simulink library "myLib_CustomBoolean"  (R2021b)
settings: Solver=VariableStepAuto  StartTime=0.0  StopTime=10.0  RelTol=1e-3
undefined symbols (not defined in the file or in its folder): get, gray, res
libraries: dspobslib x1
settings Model: Creator=abayles  LastModifiedBy=matt
settings SolverCC: AlgebraicLoopSolver=TrustRegion
settings DebuggingCC: SFMachineParentedDataDiag=warning

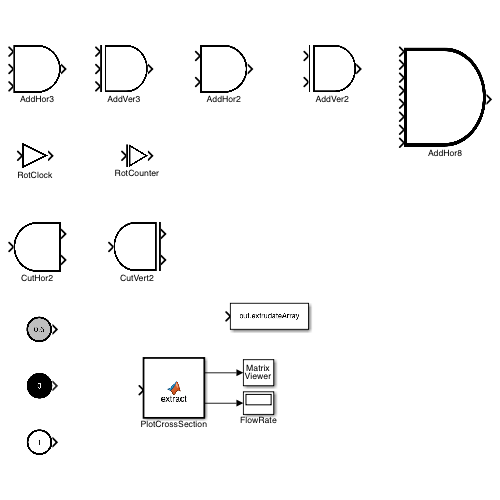
[thumbnail: Simulink's stored preview of the top-level diagram]
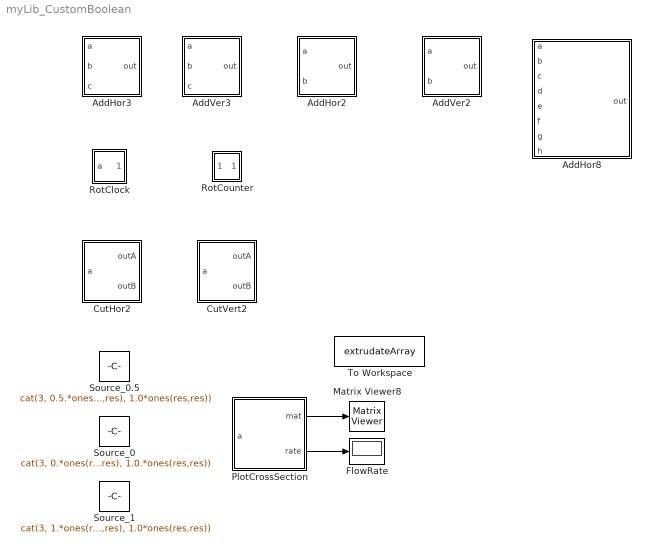
== system myLib_CustomBoolean ==
  AddHor2 : MATLAB Function  TreatAsAtomicUnit=on
  AddHor3 : MATLAB Function  TreatAsAtomicUnit=on
  AddHor8 : MATLAB Function  TreatAsAtomicUnit=on
  AddVer2 : MATLAB Function  TreatAsAtomicUnit=on
  AddVer3 : MATLAB Function  TreatAsAtomicUnit=on
  CutHor2 : MATLAB Function  TreatAsAtomicUnit=on
  CutVert2 : MATLAB Function  TreatAsAtomicUnit=on
  FlowRate : Display
  Matrix Viewer8 : dspobslib/Matrix Viewer  ImageParams=off  CMapStr=gray(3)  AxisColorbar=on  AxisParams=off  AxisOrigin=Upper left corner  AxisTickMode=User-defined  XTickRange=[0 1]  YTickRange=[0 1]  XLabel=X-axis  YLabel=Y-axis  ZLabel=Z-axis  FigPos=get(0,'defaultfigureposition')  AxisZoom=off
      settings: SourceProductBaseCode=DS  YMin=0  YMax=1
  PlotCrossSection : MATLAB Function  TreatAsAtomicUnit=on
  RotClock : MATLAB Function  TreatAsAtomicUnit=on
  RotCounter : MATLAB Function  TreatAsAtomicUnit=on
  Source_0 : Constant  Value=cat(3, 0.*ones(res,res), 1.0.*ones(res,res))  VectorParams1D=off
      mask Display:
      | % Use "Edit Image" on toolstrip to change.
      | % Insert file path below.
      | image('/Users/matt/Documents/MATLAB/UD/AdvectiveAssembly_BooleanSimulink/AdvectiveAssembly_BooleanSimulink/Examples_202112/Manuscripts/Matt-Code_v20220330/PicturesForMasks/source0.png');
  Source_0.5 : Constant  Value=cat(3, 0.5.*ones(res,res), 1.0*ones(res,res))  VectorParams1D=off
      mask Display:
      | % Use "Edit Image" on toolstrip to change.
      | % Insert file path below.
      | image('/Users/matt/Documents/MATLAB/UD/AdvectiveAssembly_BooleanSimulink/AdvectiveAssembly_BooleanSimulink/Examples_202112/Manuscripts/Matt-Code_v20220330/PicturesForMasks/source0_5.png');
  Source_1 : Constant  Value=cat(3, 1.*ones(res,res), 1.0*ones(res,res))  VectorParams1D=off
      mask Display:
      | % Use "Edit Image" on toolstrip to change.
      | % Insert file path below.
      | image('/Users/matt/Documents/MATLAB/UD/AdvectiveAssembly_BooleanSimulink/AdvectiveAssembly_BooleanSimulink/Examples_202112/Manuscripts/Matt-Code_v20220330/PicturesForMasks/source1.png');
  To Workspace : ToWorkspace  VariableName=extrudateArray  SampleTime=51
  wires:
  PlotCrossSection/1(mat) -> Matrix Viewer8/1
  PlotCrossSection/2(rate) -> FlowRate/1

== matlab function myLib_CustomBoolean/AddHor2 ==
  data: a input; out output; b input
function out = add2Hor(a, b)

== matlab function myLib_CustomBoolean/AddVer2 ==
  data: a input; out output; b input
function out = add2Ver(a,b)
%% Version and general code information
%Add Vertical V 1.0 Updated 2022-04-07
% Inputs 
    % Two 3D arrays
% Outputs
    %One 3D array
    %First 2D array (out(:,:,1)) contains the pattern.
    %last element contains the flow rate (out(:,:,2)), should be a
    %constant.

%% Determining preliminary variables
resolution = size(a,1); %Calculates resolution based off of the first dimension (# of rows) of a.
numMatrices = nargin; %Determines the number of matrices based off of the number of input arguments, two.
allMat = nan(resolution,resolution, 2*numMatrices); % Determines the total 3D array size based off the provided resolution and number of matrices. For this case the dimensions are (resolution, resolution, 4).
allMat(:,:, 1:2) = a; %Assigns all the rows and columns of the 1st and 2nd third dimension of the supplied a array to allMat. The 1st and 2nd will contain the pattern and flow rate arrays respectively.
allMat(:,:, 3:4) = b; %Assigns all the rows and columns of the 1st and 2nd third dimension of the supplied b array to allMat. The 3rd and 4th will contain the pattern and flow rate arrays of b respectively.

%% Flow rate calculation
flowRate = nan(numMatrices,1); %Create an empty vector that has numMatrices in rows (2) and 1 column.

for i = 1:numMatrices % Loop from 1 to the final number of matrices two.
    flowRate(i) = allMat(1,1,2*i); % Obtains the flow rate of each entering stream. Upon each loop iteration "grab" the 1st row, 1st column, and 2*i position in the array and assign it to the i'th spot in the flow rate vector. 
end

totalFlowRate = sum(flowRate); % Calculates the total flowrate by adding all entries in the flow rate vector.

%% Constructing the pattern matrix
reduceA = imresize(a(:,:,1),[resolution*flowRate(1)/totalFlowRate, resolution],'nearest'); % Take the pattern a(:,:,1) and resize into the specified dimensions based of the fraction of total flow rate (rows) and resolution (columns). Weights each of the matrices based on their respective flow rates (flowrate(1)).  
reduceB = imresize(b(:,:,1),[resolution*flowRate(2)/totalFlowRate, resolution],'nearest'); % Take the pattern b(:,:,1) and resize into the specified dimensions based of the fraction of total flow rate (rows) and resolution (columns). Weights each of the matrices based on their respective flow rates (flowrate(2)).  
addMatrix = [reduceA; reduceB]; % Vertically concatenates the matrices together.
addMatrix = imresize(addMatrix,[resolution, resolution],'nearest'); %Resize the image to the desired resolution dimensions. 
%% Predefining output variables
out = a; %Assigns the correct dimensions for the output variable.
out(:,:,1) = addMatrix; %Assigns the added pattern array to the output variable.
out(:,:,2) = totalFlowRate.*ones(resolution,resolution); %Defines the flow rate 2D array out(:,:,2). Calculates the new flow rate array using the total flow rate multiplied by a ones matrix of size based on the supplied resolution.

== matlab function myLib_CustomBoolean/AddHor8 ==
  data: a input; out output; b input; c input; d input; e input; f input; g input; h input
function out = add8Hor(a,b,c,d,e,f,g,h)
%% Version and general code information
%Horizontal Addition V 1.0 Updated 2022-04-07
% Inputs
    %Eight 3D arrays
% Outputs
    %3D array 
    % First 2D array (out(:,:,1)) contains the pattern
    %Last element (out(:,:,2)) contains the flow rates, should be a
    %constant

%% Determine preliminary variabes
resolution = size(a,1); %Calculates resolution based off of the first dimension (# of rows) of a
numMatrices = nargin; %Determines the number of matrices based off of the number of input arguments, eight.
allMat = nan(resolution,resolution, 2*numMatrices); % Determines the total 3D array size based off the provided resolution and number of matrices. For this case the dimensions are (resolution, resolution, 16).
allMat(:,:, 1:2) = a; %Assigns all the rows and columns of the 1st and 2nd third dimension of the supplied a array to allMat. The 1st and 2nd will contain the pattern and flow rate arrays of a respectively.
allMat(:,:, 3:4) = b; %Assigns all the rows and columns of the 1st and 2nd third dimension of the supplied b array to allMat. The 3rd and 4th will contain the pattern and flow rate arrays of b respectively.
allMat(:,:, 5:6) = c; %Assigns all the rows and columns of the 1st and 2nd third dimension of the supplied c array to allMat. The 5th and 6th will contain the pattern and flow rate arrays of c respectively.
allMat(:,:, 7:8) = d; %Assigns all the rows and columns of the 1st and 2nd third dimension of the supplied d array to allMat. The 7th and 8th will contain the pattern and flow rate arrays of d respectively.
allMat(:,:, 9:10) = e; %Assigns all the rows and columns of the 1st and 2nd third dimension of the supplied e array to allMat. The 9th and 10th will contain the pattern and flow rate arrays of e respectively.
allMat(:,:, 11:12) = f; %Assigns all the rows and columns of the 1st and 2nd third dimension of the supplied f array to allMat. The 11th and 12th will contain the pattern and flow rate arrays of f respectively.
allMat(:,:, 13:14) = g; %Assigns all the rows and columns of the 1st and 2nd third dimension of the supplied g array to allMat. The 11th and 12th will contain the pattern and flow rate arrays of g respectively.
allMat(:,:, 15:16) = h; %Assigns all the rows and columns of the 1st and 2nd third dimension of the supplied a array to allMat. The 15th and 16th will contain the pattern and flow rate arrays of h respectively.

%% Flow rate calculation
flowRate = nan(numMatrices,1); %Create an empty vector that has numMatrices in rows (8) and 1 column.
for i = 1:numMatrices % Loop from 1 to the final number of matrices 8.
    flowRate(i) = allMat(1,1,2*i); % Obtains the flow rate of each entering stream. Upon each loop iteration "grab" the 1st row, 1st column, and 2*i position in the array and assign it to the i'th spot in the flow rate vector. 
end
totalFlowRate = sum(flowRate); % Calculates the total flowrate by adding all entries in the flow rate vector.
%% Constructing the combined pattern matrix
reduceA = imresize(a(:,:,1),[resolution,resolution*flowRate(1)/totalFlowRate],'nearest'); % Take the pattern a(:,:,1) and resize into the specified dimensions based of the fraction of total flow rate (rows) and resolution (columns). Weights each of the matrices based on their respective flow rates (flowrate(1)).  
reduceB = imresize(b(:,:,1),[resolution,resolution*flowRate(2)/totalFlowRate],'nearest'); % Take the pattern b(:,:,1) and resize into the specified dimensions based of the fraction of total flow rate (rows) and resolution (columns). Weights each of the matrices based on their respective flow rates (flowrate(2)).  
reduceC = imresize(c(:,:,1),[resolution,resolution*flowRate(3)/totalFlowRate],'nearest'); % Take the pattern c(:,:,1) and resize into the specified dimensions based of the fraction of total flow rate (rows) and resolution (columns). Weights each of the matrices based on their respective flow rates (flowrate(3)).  
reduceD = imresize(d(:,:,1),[resolution,resolution*flowRate(4)/totalFlowRate],'nearest'); % Take the pattern d(:,:,1) and resize into the specified dimensions based of the fraction of total flow rate (rows) and resolution (columns). Weights each of the matrices based on their respective flow rates (flowrate(4)).  
reduceE = imresize(e(:,:,1),[resolution,resolution*flowRate(5)/totalFlowRate],'nearest'); % Take the pattern e(:,:,1) and resize into the specified dimensions based of the fraction of total flow rate (rows) and resolution (columns). Weights each of the matrices based on their respective flow rates (flowrate(5)).  
reduceF = imresize(f(:,:,1),[resolution,resolution*flowRate(6)/totalFlowRate],'nearest'); % Take the pattern f(:,:,1) and resize into the specified dimensions based of the fraction of total flow rate (rows) and resolution (columns).  Weights each of the matrices based on their respective flow rates (flowrate(6)).  
reduceG = imresize(g(:,:,1),[resolution,resolution*flowRate(7)/totalFlowRate],'nearest'); % Take the pattern g(:,:,1) and resize into the specified dimensions based of the fraction of total flow rate (rows) and resolution (columns). Weights each of the matrices based on their respective flow rates (flowrate(7)).  
reduceH = imresize(h(:,:,1),[resolution,resolution*flowRate(8)/totalFlowRate],'nearest'); % Take the pattern h(:,:,1) and resize into the specified dimensions based of the fraction of total flow rate (rows) and resolution (columns). Weights each of the matrices based on their respective flow rates (flowrate(8)).  


addMatrix = [reduceH,reduceG,reduceF,reduceE, reduceD,reduceC, reduceB, reduceA]; % Horizontally concatenates the matrices together. The point of view is from the perspective of the extrudate.
addMatrix = imresize(addMatrix,[resolution, 2.*resolution],'nearest'); %Resize the image to the desired resolution dimensions. 


%% Predefining output variables

out = [a,a]; %Assigns the correct dimensions for the output variable.
 
out(:,:,1) = addMatrix; %Assigns the added pattern array to the output variable.
out(:,:,2) = totalFlowRate.*ones(resolution,2.*resolution); %Defines the flow rate 2D array out(:,:,2). Calculates the new flow rate array using the total flow rate multiplied by a ones matrix of size based on the supplied resolution.

== matlab function myLib_CustomBoolean/RotClock ==
  data: a input; out output
function out = rotClock(a)
%% Version and general code information. 
%Rotating Clockwise Block V 1.0 Updated 2022-04-07
% Inputs:
    %3D array with pattern a(:,:,1) and flow rate a(:,:2)
%Outputs:
    %3D array
            %First 2D array (i.e., out(:,:,1)) contains the pattern
            %Last element contains the flow rate (i.e. out(:,:,2)), should be a
            %constant value.
%% Determine preliminary variables
resolution = size(a,1); %Calculates resolution based off of the first dimension (# of rows) of a.

%% Predefining output variables
out = a; %Assigns the correct dimensions for the output variable
out(:,:,1) = rot90(rot90(rot90(a(:,:,1)))); %Rotates the pattern array (a(:,:,1)) 270 degrees counterclockwise ---> 90 degrees clockwise
out(:,:,2) = a(1,1,2).*ones(resolution,resolution); % Defines the flow rate 2D array a(:,:,2)

== matlab function myLib_CustomBoolean/RotCounter ==
  data: a input; out output
function out = rotCounter(a)
%% Version and general code information
%Rotating Counter Clockwise V 1.0 Updated 2022-31-3
% Inputs:
    %3D array with pattern a(:,:,1) and flow rate a(:,:2)
%Outputs:
    %3D array
        %First 2D array (i.e., out(:,:,1)) contains the pattern
        %Last element contains the flow rate (i.e. out(:,:,2)), should be a
        %constant value.
%% Determining prelminary variables
resolution = size(a,1); %Calculates resolution based off of the first dimension (# of rows) of a.

%% Predefining output variables
out = a; %Assigns the correct dimensions for the output variable
out(:,:,1) = rot90(a(:,:,1)); % Rotates the pattern array a(:,:,1)90 degrees counterclockwise
out(:,:,2) = a(1,1,2).*ones(resolution,resolution); % Defines the flow rate 2D array a(:,:,2)

== matlab function myLib_CustomBoolean/AddHor3 ==
  data: a input; out output; b input; c input
function out = add3Hor(a, b, c)

== matlab function myLib_CustomBoolean/CutHor2 ==
  data: a input; outA output; outB output
function [outA, outB] = cutHor(a)
%% Version and general code information
%Cut Horizontal V 1.0 Updated 2022-04-07
% Inputs 
    % One 3D array
% Outputs
    %Two 3D arrays
    %First 2D array (out(:,:,1)) contains the pattern.
    %last element contains the flow rate (out(:,:,2)), should be a
    %constant.

%% Determining preliminary variables
resolution = size(a,1); %Calculates resolution based off of the first dimension (# of rows) of a.
numMatrices = nargin; %Calculates the number of matrices based off  the supplied input arguments, one. 
numOutMatrices = nargout;  %Determines the number of output matrices based off the number of output arguments,two.

%% Flow rate calculation
inputFlowRate = a(1,1,2); %Determines the inlet flow rate based off of the first element in the second 2D array of the inlet stream. 
flowRate = nan(numOutMatrices,1); % Form a vector of NaN values (2,1).

for i = 1:numOutMatrices % Loop from 1 to the final number of matrices 2.
    flowRate(i) = inputFlowRate/numOutMatrices; % Determine the new flow rate of the outlet streams based of the total inlet flow rate and number of outlet matrices (two). Store the flow rate after each iteration. Assigns equal flow rate to each stream.
end

%% Constructing the pattern matrices
cutA = imresize(a(:,1:resolution/numOutMatrices,1), [resolution, resolution],'nearest'); %Take the pattern matrix a(:,:,1) and extract all the rows, and those columns specified from to resolution/numOutMatrices. Resize this to the desired resolution based off the provided input variables.
cutB = imresize(a(:,resolution/numOutMatrices+1:end,1), [resolution, resolution],'nearest'); %Take the pattern matrix a(:,:,1) and extract all the rows and those columns from one index higher than resolution/numOutMatrices to the end of the array. Resize this to the desired resolution based off the provided input variables.

%% Predefining output variables
outA = a; %Assigns the correct dimensions for the output variable.
outB = a; %Assigns the correct dimensions for the output variable.

outA(:,:,1) = cutA; %The new pattern of array A (outA(:,:,1)) after the horizontal splitting. 
outA(:,:,2) = flowRate(1).*ones(resolution,resolution); %The new flow rate of array A (outA(:,:,2)) after the horizontal splitting. Calculates the new flow rate array using the individual flow rates (flowrate(1), first element in the flow rate vector) multiplied by a ones matrix of size based on the supplied resolution.
outB(:,:,1) = cutB; %The new pattern of array B (outB(:,:,1)) after the horizontal splitting.
outB(:,:,2) = flowRate(2).*ones(resolution,resolution); %The new flow rate of array B (outB(:,:,2)) after the horizontal splitting. Calculates the new flow rate array using the individual flow rates (flowrate(2), second element in the flow rate vector) multiplied by a ones matrix of size based on the supplied resolution.

== matlab function myLib_CustomBoolean/AddVer3 ==
  data: a input; out output; b input; c input
function out = add3Ver(a,b,c)
%% Version and general code information
%Add Vertical V 1.0 Updated 2022-04-07
% Inputs 
    % Three 3D arrays
% Outputs
    %One 3D arrays
    %First 2D array (out(:,:,1)) contains the pattern.
    %last element contains the flow rate (out(:,:,2)), should be a
    %constant.

%% Determining preliminary variables
resolution = size(a,1); %Calculates resolution based off of the first dimension (# of rows) of a.
numMatrices = nargin; %Determines the number of matrices based off of the number of input arguments, three.
allMat = nan(resolution,resolution, 2*numMatrices); % Determines the total 3D array size based off the provided resolution and number of matrices. For this case the dimensions are (resolution, resolution, 6).
allMat(:,:, 1:2) = a; %Assigns all the rows and columns of the 1st and 2nd third dimension of the supplied a array to allMat. The 1st and 2nd will contain the pattern and flow rate arrays of a respectively.
allMat(:,:, 3:4) = b; %Assigns all the rows and columns of the 1st and 2nd third dimension of the supplied b array to allMat. The 3rd and 4th will contain the pattern and flow rate arrays of b respectively.
allMat(:,:, 5:6) = c; %Assigns all the rows and columns of the 1st and 2nd third dimension of the supplied c array to allMat. The 5th and 6th will contain the pattern and flow rate arrays of c respectively.

%% Flow rate calculation
flowRate = nan(numMatrices,1); %Create an empty vector that has numMatrices in rows (3) and 1 column.

for i = 1:numMatrices % Loop from 1 to the final number of matrices 3.
    flowRate(i) = allMat(1,1,2*i); % Obtains the flow rate of each entering stream. Upon each loop iteration "grab" the 1st row, 1st column, and 2*i position in the array and assign it to the i'th spot in the flow rate vector.
end
totalFlowRate = sum(flowRate); % Calculates the total flowrate by adding all entries in the flow rate vector.

%% Constructing the pattern matrix 
reduceA = imresize(a(:,:,1),[resolution*flowRate(1)/totalFlowRate, resolution],'nearest');  % Take the pattern a(:,:,1) and resize into the specified dimensions based of the fraction of total flow rate (rows) and resolution (columns). Weights each of the matrices based on their respective flow rates (flowrate(1)).  
reduceB = imresize(b(:,:,1),[resolution*flowRate(2)/totalFlowRate, resolution],'nearest');  % Take the pattern b(:,:,1) and resize into the specified dimensions based of the fraction of total flow rate (rows) and resolution (columns). Weights each of the matrices based on their respective flow rates (flowrate(2)).  
reduceC = imresize(c(:,:,1),[resolution*flowRate(3)/totalFlowRate, resolution],'nearest');  % Take the pattern c(:,:,1) and resize into the specified dimensions based of the fraction of total flow rate (rows) and resolution (columns). Weights each of the matrices based on their respective flow rates (flowrate(3)).  
addMatrix = [reduceA; reduceB; reduceC]; % Vertically concatenates the matrices together. 
addMatrix = imresize(addMatrix,[resolution, resolution],'nearest'); %Resize the image to the desired resolution dimensions. 

%% Predefining output variables
out = a;  %Assigns the correct dimensions for the output variable.
out(:,:,1) = addMatrix; %Assigns the added pattern array to the output variable.
out(:,:,2) = totalFlowRate.*ones(resolution,resolution);  %Defines the flow rate 2D array out(:,:,2). Calculates the new flow rate array using the total flow rate multiplied by a ones matrix of size based on the supplied resolution.

== matlab function myLib_CustomBoolean/PlotCrossSection ==
  data: a input; mat output; rate output
function [mat,rate]=   extract(a)
%% Version and general code information
%Plot Cross Section V.10 Updated 2022-04-11
%Inputs
    %One 3D array
%Outputs
    %Two arrays
    % mat contains the pattern matrix a(:,:,1)
    %rate contains the total flow rate a(1,1,2)
%% Output variables
mat = double(a(:,:,1)); % The pattern matrix. Take all the rows and columns of the first 3rd dimension and assign them to the variable mat. 
rate = a(1,1,2); % The flow rate constant value. Take the first element of the second third dimension and assign it to the variable rate.

== matlab function myLib_CustomBoolean/CutVert2 ==
  data: a input; outA output; outB output
function [outA, outB] = cutVer(a)
%% Version and general code information
%Cut Vertical V 1.0 Updated 2022-04-07
% Inputs 
    % One 3D array
% Outputs
    %Two 3D arrays
    %First 2D array (out(:,:,1)) contains the pattern.
    %last element contains the flow rate (out(:,:,2)), should be a
    %constant.

%% Determining preliminary variables
resolution = size(a,1); %Calculates resolution based off of the first dimension (# of rows) of a.
numMatrices = nargin; %Calculates the number of matrices based off  the supplied input arguments, one. 
numOutMatrices = nargout; %Determines the number of output matrices based off the number of output arguments,two.

%% Flow rate calculation
inputFlowRate = a(1,1,2); %Determines the inlet flow rate based off of the first element in the second 2D array of the inlet stream. 
flowRate = nan(numOutMatrices,1); % Form a vector of NaN values (2,1).

for i = 1:numOutMatrices % Loop from 1 to the final number of matrices 2.
    flowRate(i) = inputFlowRate/numOutMatrices; % Determine the new flow rate of the outlet streams based off the total inlet flow rate and number of outlet matrices (two). Store the flow rate after each iteration. Assigns equal flow rate to each stream.
end


cutA = imresize(a(1:resolution/numOutMatrices,:,1), [resolution, resolution],'nearest'); % Take the pattern matrix a(:,:,1) and extract the first row to the row specified by resolution/numOutMatrices and all the columns. Resize this to the desired resolution based off the provided input variables.
cutB = imresize(a(resolution/numOutMatrices+1:end,:,1), [resolution, resolution],'nearest'); % Take the pattern matrix a(:,:,1) and extract the from the row specified by resoltion/numOutMatries to the last row in the matrix and all the columns. Resize this to the desired resolution based off the provided input variables.

%% Predefining output variables
outA = a; %Assigns the correct dimensions for the output variable.
outB = a; %Assigns the correct dimensions for the output variable.

outA(:,:,1) = cutA; %The new pattern of array A (outA(:,:,1)) after the vertical splitting. 
outA(:,:,2) = flowRate(1).*ones(resolution,resolution); %The new flow rate of array A (outA(:,:,2)) after the horizontal splitting. Calculates the new flow rate array using the individual flow rates (flowrate(1), first element in the flow rate vector) multiplied by a ones matrix of size based on the supplied resolution.
outB(:,:,1) = cutB; %The new pattern of array B (outB(:,:,1)) after the vertical splitting.
outB(:,:,2) = flowRate(2).*ones(resolution,resolution); %The new flow rate of array B (outB(:,:,2)) after the horizontal splitting. Calculates the new flow rate array using the individual flow rates (flowrate(2), second element in the flow rate vector) multiplied by a ones matrix of size based on the supplied resolution.
